simulink model "untitled_v2_update"  (R2025b)
settings: Solver=VariableStepAuto  StartTime=0.0  StopTime=10  RelTol=1e-3
PreLoadFcn:
  | load('AEB_configure.mat')
undefined symbols (not defined in the file): d_min, m, rwh, Tbr_max
libraries: slpidlib x1
settings Model: Creator=duyba

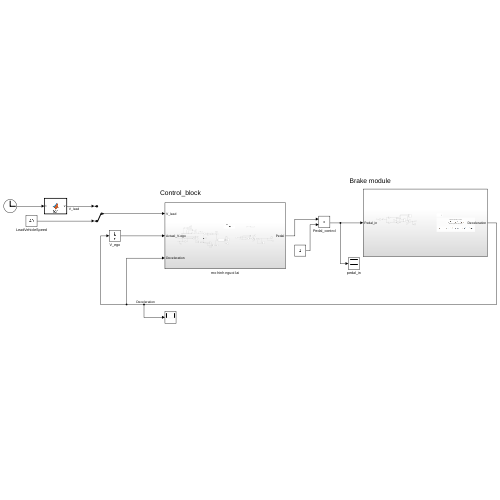
[thumbnail: Simulink's stored preview of the top-level diagram]
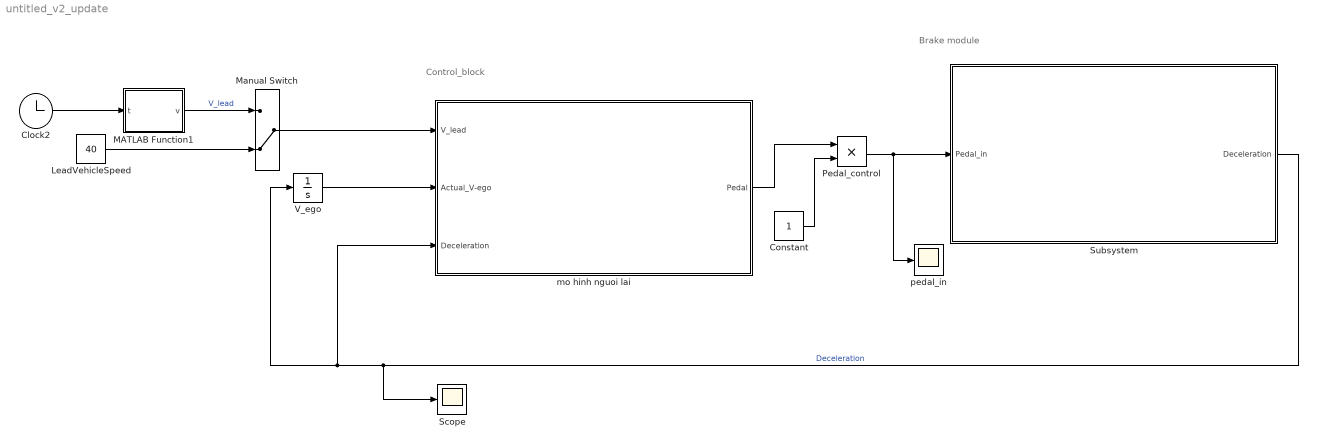
== system untitled_v2_update ==
  note: Control_block
  note: Brake module
  Clock2 : Clock
  Constant : Constant
  LeadVehicleSpeed : Constant  Value=40
  MATLAB Function1 : MATLAB Function  TreatAsAtomicUnit=on
  Manual Switch : ManualSwitch  CurrentSetting=0
  Pedal_control : Product
  Scope : Scope
      settings: ActiveDisplayYMinimum=-8.916530956689364  ActiveDisplayYMaximum=-8.2107755384854535  DataLoggingVariableName=ScopeData2
  Subsystem : Subsystem
  V_ego : Integrator  InitialCondition=60
  mo hinh nguoi lai : Subsystem
  pedal_in : Scope
      settings: ActiveDisplayYMinimum=-1.1842806749496004  ActiveDisplayYMaximum=1.3767676467994066  DataLoggingVariableName=ScopeData8
  wires:
  mo hinh nguoi lai/1(Pedal) -> Pedal_control/1
  LeadVehicleSpeed/1 -> Manual Switch/2
  MATLAB Function1/1(v) -> Manual Switch/1  "V_lead"
  Clock2/1 -> MATLAB Function1/1(t)
  Manual Switch/1 -> mo hinh nguoi lai/1(V_lead)
  Subsystem/1(Deceleration) -> Scope/1, mo hinh nguoi lai/3(Deceleration), V_ego/1  "Deceleration"
  V_ego/1 -> mo hinh nguoi lai/2(Actual_V-ego)
  Pedal_control/1 -> pedal_in/1, Subsystem/1("Pedal_in ")
  Constant/1 -> Pedal_control/2

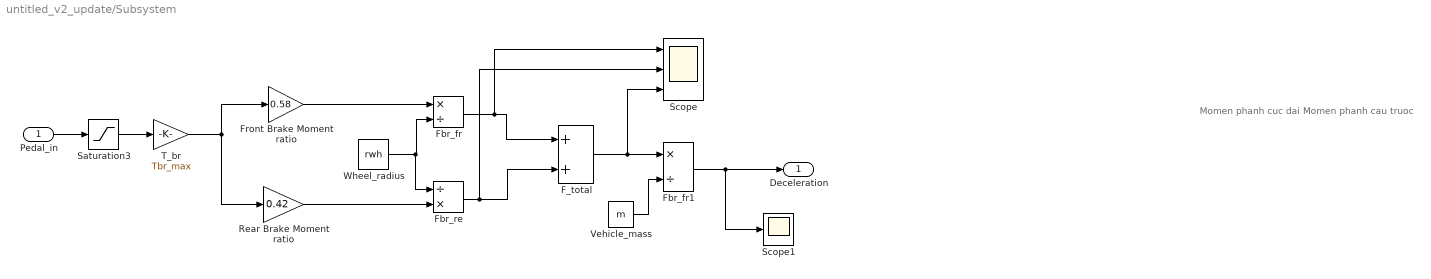
== system untitled_v2_update/Subsystem ==
  note: Momen phanh cuc dai
      |
      | Momen phanh cau truoc
  "Pedal_in " : Inport
  F_total : Sum
  Fbr_fr : Product  Inputs=*/
  Fbr_fr1 : Product  Inputs=*/
  Fbr_re : Product  Inputs=/*
  Front Brake Moment ratio : Gain  Gain=0.58  SaturateOnIntegerOverflow=on  OutDataTypeStr=Inherit: Same as input  ParamDataTypeStr=Inherit: Same as input
  Rear Brake Moment ratio : Gain  Gain=0.42  SaturateOnIntegerOverflow=on  OutDataTypeStr=Inherit: Same as input  ParamDataTypeStr=Inherit: Same as input
  Saturation3 : Saturate  UpperLimit=0  LowerLimit=-1
  Scope : Scope  NumInputPorts=3
      settings: ActiveDisplayYMinimum=-5447.851800661746  ActiveDisplayYMaximum=4650.4865483241092
  Scope1 : Scope
      settings: ActiveDisplayYMinimum=-9.6041074099695081  ActiveDisplayYMaximum=-6.97885753502311  DataLoggingVariableName=ScopeData6
  T_br : Gain  Gain=Tbr_max  SaturateOnIntegerOverflow=on  OutDataTypeStr=Inherit: Same as input  ParamDataTypeStr=Inherit: Same as input
  Vehicle_mass : Constant  Value=m
  Wheel_radius : Constant  Value=rwh
  Deceleration : Outport
  wires:
  "Pedal_in "/1 -> Saturation3/1
  Saturation3/1 -> T_br/1
  T_br/1 -> Rear Brake Moment ratio/1, Front Brake Moment ratio/1
  Front Brake Moment ratio/1 -> Fbr_fr/1
  Wheel_radius/1 -> Fbr_re/1, Fbr_fr/2
  Rear Brake Moment ratio/1 -> Fbr_re/2
  Fbr_fr/1 -> Scope/1, F_total/1
  Fbr_re/1 -> Scope/2, F_total/2
  F_total/1 -> Scope/3, Fbr_fr1/1
  Vehicle_mass/1 -> Fbr_fr1/2
  Fbr_fr1/1 -> Scope1/1, Deceleration/1

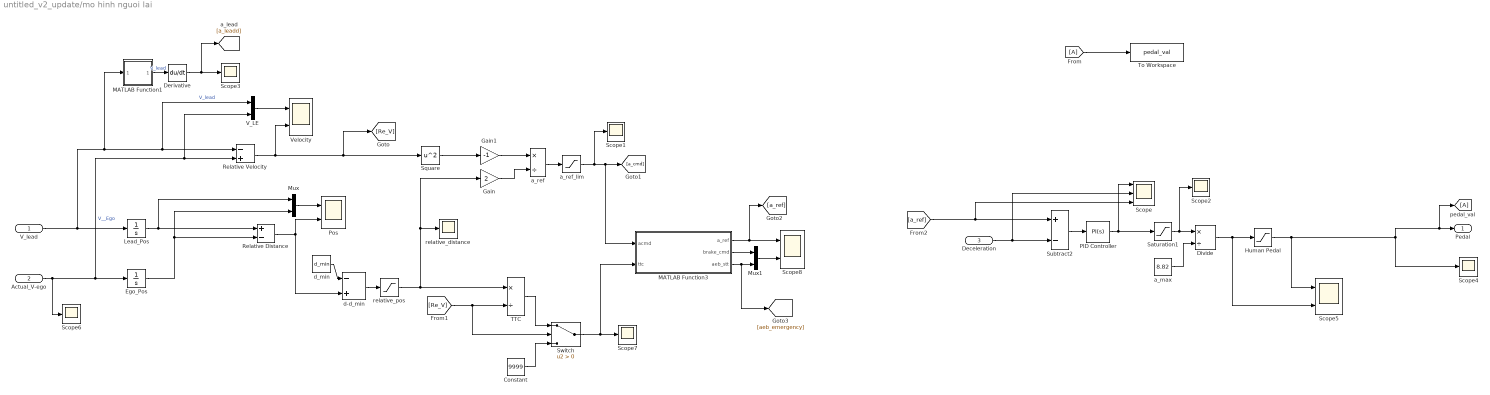
== system untitled_v2_update/mo hinh nguoi lai ==
  V_lead : Inport
  Actual_V-ego : Inport  Port=2
  Deceleration : Inport  Port=3
  Constant : Constant  Value=9999
  Derivative : Derivative
  Divide : Product  Inputs=*/
  Ego_Pos : Integrator
  From : From
  Gain : Gain  Gain=2
  Gain1 : Gain  Gain=-1
  Human Pedal : Saturate  UpperLimit=0  LowerLimit=-1
  Lead_Pos : Integrator  InitialCondition=50
  MATLAB Function1 : MATLAB Function  TreatAsAtomicUnit=on
  MATLAB Function3 : MATLAB Function  TreatAsAtomicUnit=on
  Mux : Mux  Inputs=2
  Mux1 : Mux  Inputs=2
  PID Controller : slpidlib/PID Controller  Controller=PI  Form=Parallel  TimeDomain=Continuous-time  UseExternalTs=off  SampleTime=-1  IntegratorMethod=Forward Euler  FilterMethod=Forward Euler  ControllerParametersSource=internal  P=6  I=4  UseKiTs=off  D=0  UseExternalDerivativeSource=off  N=10  UseFilter=on  TunerSelectOption=Transfer Function Based (PID Tuner App)  InitialConditionSource=internal  InitialConditionForIntegrator=0  InitialConditionForFilter=0  DifferentiatorICPrevScaledInput=0  ExternalReset=none  TrackingMode=off  Kt=1  LimitOutput=off  SatLimitsSource=internal  UpperSaturationLimit=inf  LowerSaturationLimit=-inf  LinearizeAsGain=on  AntiWindupMode=none  Kb=1  LimitIntegrator=off  UpperIntegratorSaturationLimit=inf  LowerIntegratorSaturationLimit=-inf  POutMin=[]  POutMax=[]  IOutMin=[]  IOutMax=[]  DOutMin=[]  DOutMax=[]  NOutMin=[]  NOutMax=[]  SumOutMin=[]  SumOutMax=[]  SaturationOutMin=[]  SaturationOutMax=[]  PParamMin=[]  PParamMax=[]  IParamMin=[]  IParamMax=[]  DParamMin=[]  DParamMax=[]  NParamMin=[]  NParamMax=[]  KbParamMin=[]  KbParamMax=[]  KtParamMin=[]  KtParamMax=[]  KbOutMin=[]  KbOutMax=[]  KtOutMin=[]  KtOutMax=[]  IntegratorOutMin=[]  IntegratorOutMax=[]  FilterOutMin=[]  FilterOutMax=[]  SumI1OutMin=[]  SumI1OutMax=[]  SumI2OutMin=[]  SumI2OutMax=[]  SumI3OutMin=[]  SumI3OutMax=[]  SumI4OutMin=[]  SumI4OutMax=[]  SumDOutMin=[]  SumDOutMax=[]  DifferentiatorOutMin=[]  DifferentiatorOutMax=[]  FilterDiffOutCoefMin=[]  FilterDiffOutCoefMax=[]  ReciprocalOutMin=[]  ReciprocalOutMax=[]  SumDenOutMin=[]  SumDenOutMax=[]  SumNumOutMin=[]  SumNumOutMax=[]  DivideOutMin=[]  DivideOutMax=[]  UdiffTsProdOutMin=[]  UdiffTsProdOutMax=[]  NTsProdOutMin=[]  NTsProdOutMax=[]  UintegralTsProdOutMin=[]  UintegralTsProdOutMax=[]  UngainTsProdOutMin=[]  UngainTsProdOutMax=[]  ClampingZeroOutDataTypeStr=Inherit: Inherit via back propagation  ClampingZeroOutMin=[]  ClampingZeroOutMax=[]  FilterDenConstantOutDataTypeStr=Inherit: Inherit via back propagation  FilterDenConstantOutMin=[]  FilterDenConstantOutMax=[]  PCopyOutDataTypeStr=Inherit: Inherit via back propagation  PCopyOutMin=[]  PCopyOutMax=[]  NCopyOutDataTypeStr=Inherit: Inherit via back propagation  NCopyOutMin=[]  NCopyOutMax=[]  IntegratorContinuousStateAttributes=''  IntegratorStateMustResolveToSignalObject=off  IntegratorRTWStateStorageClass=Auto  FilterContinuousStateAttributes=''  FilterStateMustResolveToSignalObject=off  FilterRTWStateStorageClass=Auto  ParallelPVariant=InternalParameters  IdealPVariant=Disabled  IVariant=InternalParameters  DVariant=Disabled  IntegratorVariant=Continuous  SatVariant=Disabled  AWVariant=Passthrough  PCopyVariant=Disabled  TRVariant=Disabled  FdbkBlocksVariant=Forward  IdealPFdbkVariant=Disabled  SatFdbkVariant=Disabled  DerivativeFilterVariant=Disabled  NVariant=Disabled  NCopyVariant=Disabled_SignalSpec  FilterICVariant=Disabled  IntegratorICVariant=InternalICs  ExternalResetVariant=Disabled  TRSumVariant=Passthrough  SumFdbkVariant=Disabled  SumVariant=Sum_PI  TsampFilterVariant=InternalTs  TsampNgainVariant=Passthrough  TsampIntegralVariant=Disabled_SignalSpec  ExternalSaturationOutDataTypeStr=Inherit: Same as second input  DerivativeSourceVariant=Disabled  PreIntVariant=InternalPreInt
  Pos : Scope  NumInputPorts=2
      settings: ActiveDisplayYMinimum=-225.38055690976771  ActiveDisplayYMaximum=501.54893996101163  DataLoggingVariableName=ScopeData4
  Relative Distance : Sum  Inputs=+-
  Relative Velocity : Sum  Inputs=-+
  Saturation1 : Saturate  UpperLimit=0  LowerLimit=-9.81
  Scope : Scope  NumInputPorts=3
      settings: ActiveDisplayYMinimum=-14.26036745156375  ActiveDisplayYMaximum=7.048587398036366  DataLoggingVariableName=ScopeData3
  Scope{1..4,6..7} (6 alike) : Scope
      Scope1 settings: ActiveDisplayYMinimum=-21.930403196042693  ActiveDisplayYMaximum=16.082631658758441  DataLoggingVariableName=ScopeData13
      Scope2 settings: ActiveDisplayYMinimum=-14.42338319151558  ActiveDisplayYMaximum=7.0717807136366382  DataLoggingVariableName=ScopeData5
      Scope3 settings: ActiveDisplayYMinimum=-11.809487971743977  ActiveDisplayYMaximum=6.01939244441855  DataLoggingVariableName=ScopeData7
      Scope4 settings: ActiveDisplayYMinimum=-1.2967421440982185  ActiveDisplayYMaximum=0.3394467683583946  DataLoggingVariableName=ScopeData10
      Scope6 settings: ActiveDisplayYMinimum=39.87906296713571  ActiveDisplayYMaximum=75.367379759772874  DataLoggingVariableName=ScopeData11
      Scope7 settings: ActiveDisplayYMinimum=-6.7809069921150638  ActiveDisplayYMaximum=36.594778865196034  DataLoggingVariableName=ScopeData14
  Scope5 : Scope  NumInputPorts=2
      settings: ActiveDisplayYMinimum=-8144.0876709405311  ActiveDisplayYMaximum=3416.5190298861144  DataLoggingVariableName=ScopeData9
  Scope8 : Scope  NumInputPorts=2
      settings: ActiveDisplayYMinimum=-15.309061672094604  ActiveDisplayYMaximum=4.315380835297816  DataLoggingVariableName=ScopeData15
  Square : Math  Operator=square
  Subtract2 : Sum  Inputs=+-
  Switch : Switch  Criteria=u2 > Threshold  SaturateOnIntegerOverflow=off  InputSameDT=off
  TTC : Product  Inputs=*/
  To Workspace : ToWorkspace  VariableName=pedal_val  SaveFormat=Timeseries  SampleTime=-1
  V_LE : Mux  Inputs=2
  Velocity : Scope  NumInputPorts=2
      settings: ActiveDisplayYMinimum=23.505192207596412  ActiveDisplayYMaximum=102.84777896960448
  a_max : Constant  Value=8.82
  a_ref : Product  Inputs=*/
  a_ref_lim : Saturate  UpperLimit=0  LowerLimit=-9.8
  d-d_min : Sum  Inputs=-+
  d_min : Constant  Value=d_min
  pedal_val : Goto
  relative_distance : Scope
      settings: ActiveDisplayYMinimum=-46.488813562071073  ActiveDisplayYMaximum=185.40903525270232  DataLoggingVariableName=ScopeData12
  relative_pos : Saturate  UpperLimit=9999  LowerLimit=0.1
  Pedal : Outport
  wires:
  PID Controller/1 -> Saturation1/1, Scope/1
  Subtract2/1 -> PID Controller/1
  Ego_Pos/1 -> Mux/2, Relative Distance/2
  Relative Distance/1 -> d-d_min/2, Pos/2
  V_lead/1 -> MATLAB Function1/1(v_km), V_LE/1, Relative Velocity/1, Lead_Pos/1  "V_lead"
  Lead_Pos/1 -> Mux/1, Relative Distance/1
  Actual_V-ego/1 -> Scope6/1, V_LE/2, Relative Velocity/2, Ego_Pos/1  "V__Ego"
  Deceleration/1 -> Scope/2, Subtract2/2
  relative_pos/1 -> TTC/1, relative_distance/1, Gain/1
  Relative Velocity/1 -> [Re_V], Square/1, Velocity/2
  d_min/1 -> d-d_min/1
  Square/1 -> Gain1/1
  Gain/1 -> a_ref/2
  Gain1/1 -> a_ref/1
  a_ref/1 -> a_ref_lim/1
  d-d_min/1 -> relative_pos/1
  a_max/1 -> Divide/2
  Divide/1 -> Scope5/2, Human Pedal/1
  Saturation1/1 -> Scope2/1, Divide/1
  V_LE/1 -> Velocity/1
  From/1 -> To Workspace/1
  Derivative/1 -> [a_leadd], Scope3/1
  MATLAB Function1/1(v_m) -> Derivative/1  "V_lead"
  Mux/1 -> Pos/1
  [a_ref] -> Scope/3, Subtract2/1
  [Re_V] -> Switch/2, TTC/2
  TTC/1 -> Switch/1
  Constant/1 -> Switch/3
  Switch/1 -> MATLAB Function3/2(ttc), Scope7/1
  a_ref_lim/1 -> MATLAB Function3/1(acmd), [a_cmd], Scope1/1
  MATLAB Function3/2(brake_cmd) -> Mux1/1
  MATLAB Function3/3(aeb_stt) -> [aeb_emergency], Mux1/2
  Mux1/1 -> Scope8/2
  MATLAB Function3/1(a_ref) -> [a_ref], Scope8/1
  Human Pedal/1 -> pedal_val/1, Pedal/1, Scope4/1, Scope5/1

== matlab function untitled_v2_update/mo hinh nguoi lai/MATLAB Function1 ==
  data: v_km input; v_m output
function v_m = fcn(v_km)
% Gia toc phanh 6 m/s^2, v0 = 50 km/h

v_m = v_km /3.6; %doi km/h -> m/s
end

== matlab function untitled_v2_update/mo hinh nguoi lai/MATLAB Function3 ==
  data: acmd input; ttc input; a_ref output; brake_cmd output; aeb_stt output
function [a_ref, brake_cmd, aeb_stt] = fcn(acmd, ttc)

%parameter setup
a_offset =2;
a_ref=0;
brake_cmd=0;
aeb_stt=0;
a_thres=2;

if (0<ttc)&& (ttc <a_thres) %full
    brake_cmd=1;
    aeb_stt=4;
    a_ref = acmd - (brake_cmd*aeb_stt*a_offset);

elseif ttc<a_thres+2 %partial 2
    brake_cmd=1; 
    aeb_stt=3;
    a_ref = acmd - (brake_cmd*aeb_stt*a_offset);

elseif ttc<a_thres+6 % partial 1
    brake_cmd=1;
    aeb_stt=2;
    a_ref = acmd - (brake_cmd*aeb_stt*a_offset);

elseif ttc<a_thres+10 %warning
    brake_cmd=0;
    aeb_stt=1;
    a_ref = acmd - (brake_cmd*aeb_stt*a_offset);
elseif ttc >= a_thres+10 %safe 
    brake_cmd=0;
    aeb_stt=0;
    a_ref =0;
end

== matlab function untitled_v2_update/MATLAB Function1 ==
  data: t input; v output
% function v = fcn(t)
% % 6m/s^2 he so bam 0.8, v = 50km/h
% function v = fcn(t)
%     if t < 2 && t >= 0
%         y = 13.89;
%     elseif t >= 2 && t < 4.35712
%         y = -(2.5) * (t-2)^2 + 13.89;
%     else
%         y = 0;
%     end
% end
%% 2m/s^2 he so bam 0.8, v = 50km/h
function v = fcn(t)
% Gia toc phanh 6 m/s^2, v0 = 50 km/h

v0 = 13.89;   % m/s
a  = -4;      % m/s^2
t0 = 2;       % thoi diem bat dau phanh

if t < t0
    v = v0;
elseif t < t0 + v0/(-a)
    v = v0 + a*(t - t0);
else
    v = 0;
end

v = v * 3.6; %doi m/s -> km/h
end
